simulink model "MathLibEasyTest"  (R2016b)
settings: Solver=VariableStepAuto  StartTime=0.0  StopTime=10.0  RelTol=1e-3
settings Model: Creator=Administrator  LastModifiedBy=Administrator

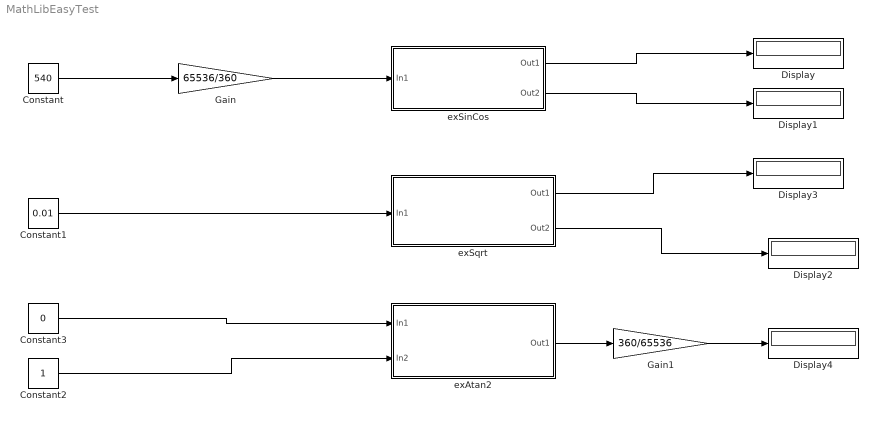
== system MathLibEasyTest ==
  Constant : Constant  Value=540  OutDataTypeStr=single
  Constant1 : Constant  Value=0.01  OutDataTypeStr=single
  Constant2 : Constant  OutDataTypeStr=single
  Constant3 : Constant  Value=0  OutDataTypeStr=single
  Display{,1..4} (5 alike) : Display
  Gain : Gain  Gain=65536/360
  Gain1 : Gain  Gain=360/65536
  exAtan2 : Subsystem
      mask help:
      | tan(theta) = yAxis/xAxis
      | theta: [0 65536) --> [0 360)
      mask Display:
      | disp('sincos in C');
      | port_label('input',1,'yAxis');
      | port_label('input',2,'xAxis');
      | port_label('output',1,'theta');
  exSinCos : Subsystem
      mask help:
      | x: [0 65536) -->[0 360)
      | sin: [-32767 32767] -->[-1 1]
      | cos: [-32767 32767] -->[-1 1]
      mask Display:
      | disp('sincos in C');
      | port_label('input',1,'x');
      | port_label('output',1,'sinx');
      | port_label('output',2,'cosx');
  exSqrt : Subsystem
      mask help: x=0 when x<0
      mask Display:
      | disp('sqrt in C');
      | port_label('input',1,'x');
      | port_label('output',1,'sqrtx');
      | port_label('output',2,'1/sqrtx');
  wires:
  Constant/1 -> Gain/1
  exSinCos/1(Out1) -> Display/1
  exSinCos/2(Out2) -> Display1/1
  Gain/1 -> exSinCos/1(In1)
  Constant1/1 -> exSqrt/1(In1)
  exSqrt/1(Out1) -> Display3/1
  exSqrt/2(Out2) -> Display2/1
  Constant3/1 -> exAtan2/1(In1)
  Constant2/1 -> exAtan2/2(In2)
  exAtan2/1(Out1) -> Gain1/1
  Gain1/1 -> Display4/1

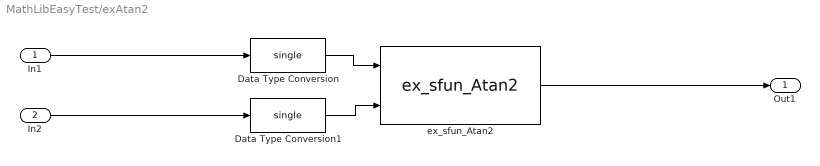
== system MathLibEasyTest/exAtan2 ==
  In1 : Inport
  In2 : Inport  Port=2
  Data Type Conversion : DataTypeConversion  OutDataTypeStr=single
  Data Type Conversion1 : DataTypeConversion  OutDataTypeStr=single
  ex_sfun_Atan2 : S-Function  FunctionName=ex_sfun_Atan2  SFunctionDeploymentMode=off  EnableBusSupport=off  mask(Legacy Function){SFunctionSpec=void Atan2Shell(single u1,single u2,uint16 y1[1]), ShowSpec=on}
      mask prompts: ShowSpec "Display function specification"
      mask help:
      | This block allows you to call the legacy functions specified by the following Legacy Code Tool definition:
      | def.SFunctionName = 'ex_sfun_Atan2';
      | def.OutputFcnSpec = 'void Atan2Shell(single u1,single u2,uint16 y1[1])';
      | def.HeaderFiles = {'C2SfunShell.h', 'typedefs.h', 'LIB_Atan2.h', 'LIB_SinCosCalc.h', 'LIB_SqrtCalc.h'};
      | def.SourceFiles = {'C2SfunShell.c', 'LIB_Atan2.c', 'LIB_SinCosCalc.c', 'LIB_SqrtCalc.c'};
      mask Help: <p>This block was generated automatically by the Legacy Code Tool. For detailed help on this tool, call<a href="matlab:legacy_code('help')"> legacy_code('help')</a>.</p>
      mask Callback ShowSpec:
      | if strcmp(get_param(gcbh, 'ShowSpec'), 'on')
      |   set_param(gcbh, 'MaskDisplay', sprintf('fprintf(''%s'');', get_param(gcbh, 'SFunctionSpec')));
      | else
      |   set_param(gcbh, 'MaskDisplay', sprintf('fprintf(''%s'');', get_param(gcbh, 'FunctionName')));
      | end
      mask Display: fprintf('void Atan2Shell(single u1,single u2,uint16 y1[1])');
  Out1 : Outport
  wires:
  Data Type Conversion1/1 -> ex_sfun_Atan2/2
  Data Type Conversion/1 -> ex_sfun_Atan2/1
  In1/1 -> Data Type Conversion/1
  ex_sfun_Atan2/1 -> Out1/1
  In2/1 -> Data Type Conversion1/1

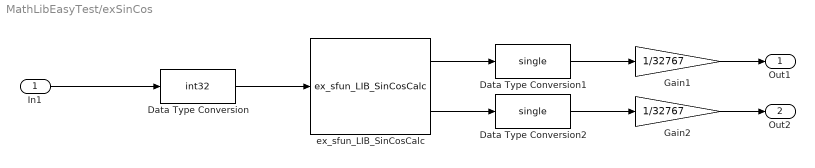
== system MathLibEasyTest/exSinCos ==
  In1 : Inport
  Data Type Conversion : DataTypeConversion  OutDataTypeStr=int32
  Data Type Conversion1 : DataTypeConversion  OutDataTypeStr=single
  Data Type Conversion2 : DataTypeConversion  OutDataTypeStr=single
  Gain1 : Gain  Gain=1/32767
  Gain2 : Gain  Gain=1/32767
  ex_sfun_LIB_SinCosCalc : S-Function  FunctionName=ex_sfun_LIB_SinCosCalc  SFunctionDeploymentMode=off  EnableBusSupport=off  mask(Legacy Function){SFunctionSpec=void SinCosShell(int32 u1,int16 y1[1],int16 y2[1]), ShowSpec=on}
      mask prompts: ShowSpec "Display function specification"
      mask help:
      | This block allows you to call the legacy functions specified by the following Legacy Code Tool definition:
      | def.SFunctionName = 'ex_sfun_LIB_SinCosCalc';
      | def.OutputFcnSpec = 'void SinCosShell(int32 u1,int16 y1[1],int16 y2[1])';
      | def.HeaderFiles = {'C2SfunShell.h', 'typedefs.h', 'LIB_Atan2.h', 'LIB_SinCosCalc.h', 'LIB_SqrtCalc.h'};
      | def.SourceFiles = {'C2SfunShell.c', 'LIB_Atan2.c', 'LIB_SinCosCalc.c', 'LIB_SqrtCalc.c'};
      mask Help: <p>This block was generated automatically by the Legacy Code Tool. For detailed help on this tool, call<a href="matlab:legacy_code('help')"> legacy_code('help')</a>.</p>
      mask Callback ShowSpec:
      | if strcmp(get_param(gcbh, 'ShowSpec'), 'on')
      |   set_param(gcbh, 'MaskDisplay', sprintf('fprintf(''%s'');', get_param(gcbh, 'SFunctionSpec')));
      | else
      |   set_param(gcbh, 'MaskDisplay', sprintf('fprintf(''%s'');', get_param(gcbh, 'FunctionName')));
      | end
      mask Display: fprintf('void SinCosShell(int32 u1,int16 y1[1],int16 y2[1])');
  Out1 : Outport
  Out2 : Outport  Port=2
  wires:
  Gain1/1 -> Out1/1
  ex_sfun_LIB_SinCosCalc/1 -> Data Type Conversion1/1
  Data Type Conversion1/1 -> Gain1/1
  Data Type Conversion/1 -> ex_sfun_LIB_SinCosCalc/1
  In1/1 -> Data Type Conversion/1
  Data Type Conversion2/1 -> Gain2/1
  Gain2/1 -> Out2/1
  ex_sfun_LIB_SinCosCalc/2 -> Data Type Conversion2/1

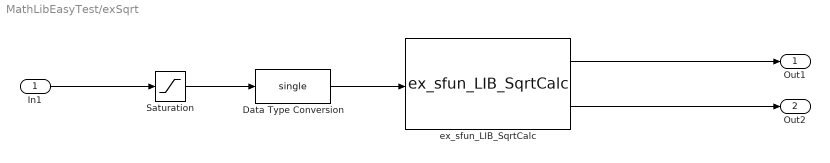
== system MathLibEasyTest/exSqrt ==
  In1 : Inport
  Data Type Conversion : DataTypeConversion  OutDataTypeStr=single
  Saturation : Saturate  UpperLimit=inf  LowerLimit=0
  ex_sfun_LIB_SqrtCalc : S-Function  FunctionName=ex_sfun_LIB_SqrtCalc  SFunctionDeploymentMode=off  EnableBusSupport=off  mask(Legacy Function){SFunctionSpec=void SqrtShell(single u1,single y1[1],single y2[1]), ShowSpec=on}
      mask prompts: ShowSpec "Display function specification"
      mask help:
      | This block allows you to call the legacy functions specified by the following Legacy Code Tool definition:
      | def.SFunctionName = 'ex_sfun_LIB_SqrtCalc';
      | def.OutputFcnSpec = 'void SqrtShell(single u1,single y1[1],single y2[1])';
      | def.HeaderFiles = {'C2SfunShell.h', 'typedefs.h', 'LIB_Atan2.h', 'LIB_SinCosCalc.h', 'LIB_SqrtCalc.h'};
      | def.SourceFiles = {'C2SfunShell.c', 'LIB_Atan2.c', 'LIB_SinCosCalc.c', 'LIB_SqrtCalc.c'};
      mask Help: <p>This block was generated automatically by the Legacy Code Tool. For detailed help on this tool, call<a href="matlab:legacy_code('help')"> legacy_code('help')</a>.</p>
      mask Callback ShowSpec:
      | if strcmp(get_param(gcbh, 'ShowSpec'), 'on')
      |   set_param(gcbh, 'MaskDisplay', sprintf('fprintf(''%s'');', get_param(gcbh, 'SFunctionSpec')));
      | else
      |   set_param(gcbh, 'MaskDisplay', sprintf('fprintf(''%s'');', get_param(gcbh, 'FunctionName')));
      | end
      mask Display: fprintf('void SqrtShell(single u1,single y1[1],single y2[1])');
  Out1 : Outport
  Out2 : Outport  Port=2
  wires:
  ex_sfun_LIB_SqrtCalc/2 -> Out2/1
  In1/1 -> Saturation/1
  ex_sfun_LIB_SqrtCalc/1 -> Out1/1
  Data Type Conversion/1 -> ex_sfun_LIB_SqrtCalc/1
  Saturation/1 -> Data Type Conversion/1
